simulink subsystem "IVTs"  (R2023b)
settings: Solver=VariableStepAuto  StartTime=0.0  StopTime=10.0  RelTol=1e-3
undefined symbols (not defined in the file): BServiceDisconnectNeg, BServiceDisconnectPos, tSimCont
settings Model: DataDictionary=Contactors_data.sldd  EnableAccessToBaseWorkspace=off  Creator=Elio  LastModifiedBy=Elio

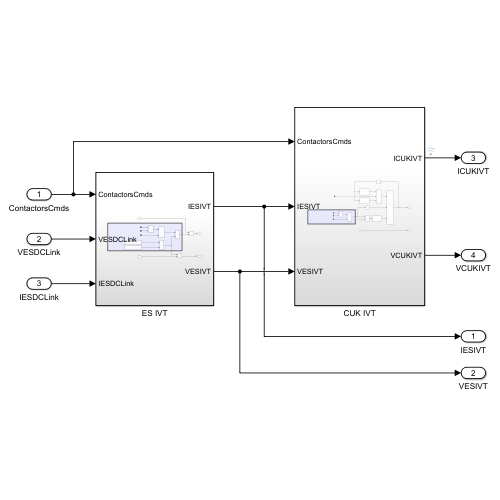
[thumbnail: Simulink's stored preview of the top-level diagram]
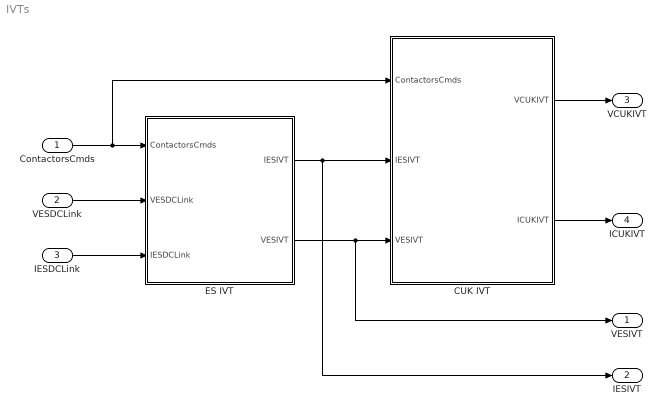
== system IVTs ==
  ContactorsCmds : Inport
  VESDCLink : Inport  Port=2
  IESDCLink : Inport  Port=3
  CUK IVT : Subsystem
  ES IVT : Subsystem
  VESIVT : Outport
  IESIVT : Outport  Port=2
  VCUKIVT : Outport  Port=3
  ICUKIVT : Outport  Port=4
  wires:
  ES IVT/1(IESIVT) -> IESIVT/1, CUK IVT/2(IESIVT)
  ES IVT/2(VESIVT) -> VESIVT/1, CUK IVT/3(VESIVT)
  CUK IVT/2(ICUKIVT) -> ICUKIVT/1
  CUK IVT/1(VCUKIVT) -> VCUKIVT/1
  ContactorsCmds/1 -> CUK IVT/1(ContactorsCmds), ES IVT/1(ContactorsCmds)
  VESDCLink/1 -> ES IVT/2(VESDCLink)
  IESDCLink/1 -> ES IVT/3(IESDCLink)

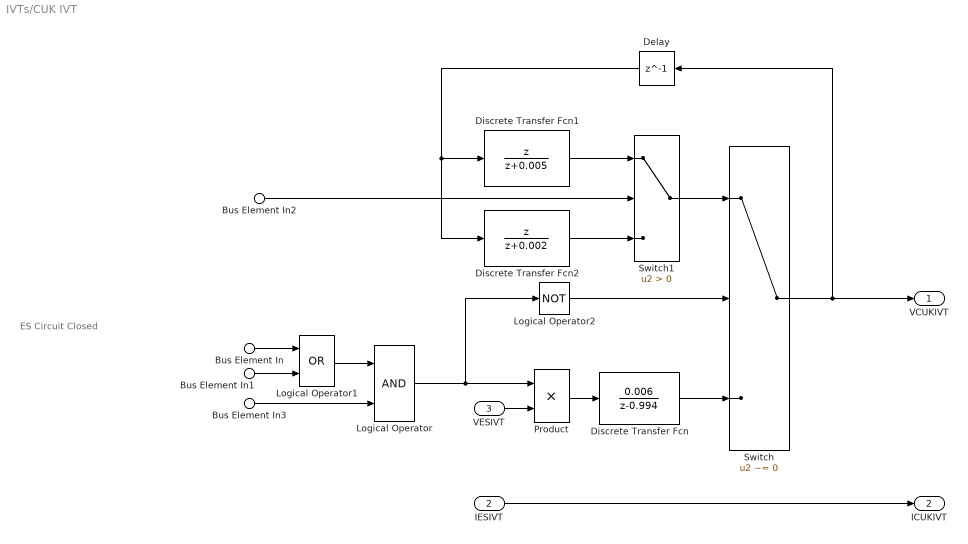
== system IVTs/CUK IVT ==
  note: ES Circuit Closed
  Bus Element In : Inport  PortName=ContactorsCmds  Element=BContPosRequested
  Bus Element In3 : Inport  PortName=ContactorsCmds  Element=BContNegRequested
  Bus Element In1 : Inport  PortName=ContactorsCmds  Element=BPrechargeRequested
  Bus Element In2 : Inport  PortName=ContactorsCmds  Element=BActiveDischargeRequested
  IESIVT : Inport  Port=2
  VESIVT : Inport  Port=3
  Delay : Delay  DelayLength=1
  Discrete Transfer Fcn : DiscreteTransferFcn  Numerator=[0.006]  Denominator=[1 -0.994]
  Discrete Transfer Fcn1 : DiscreteTransferFcn  Numerator=[1 0]  Denominator=[1 0.005]
  Discrete Transfer Fcn2 : DiscreteTransferFcn  Numerator=[1 0]  Denominator=[1 0.002]
  Logical Operator : Logic  AllPortsSameDT=off  OutDataTypeStr=boolean
  Logical Operator1 : Logic  Operator=OR  AllPortsSameDT=off  OutDataTypeStr=boolean
  Logical Operator2 : Logic  Operator=NOT  AllPortsSameDT=off  OutDataTypeStr=boolean
  Product : Product
  Switch : Switch  Criteria=u2 ~= 0  SaturateOnIntegerOverflow=off  InputSameDT=off
  Switch1 : Switch  Criteria=u2 > Threshold  SaturateOnIntegerOverflow=off  InputSameDT=off
  VCUKIVT : Outport
  ICUKIVT : Outport  Port=2
  wires:
  Switch/1 -> VCUKIVT/1, Delay/1
  Product/1 -> Discrete Transfer Fcn/1
  VESIVT/1 -> Product/2
  Bus Element In3/1 -> Logical Operator/2
  Logical Operator1/1 -> Logical Operator/1
  Bus Element In1/1 -> Logical Operator1/2
  Bus Element In/1 -> Logical Operator1/1
  Discrete Transfer Fcn/1 -> Switch/3
  Delay/1 -> Discrete Transfer Fcn1/1, Discrete Transfer Fcn2/1
  Bus Element In2/1 -> Switch1/2
  Logical Operator/1 -> Product/1, Logical Operator2/1
  Switch1/1 -> Switch/1
  Discrete Transfer Fcn1/1 -> Switch1/1
  Discrete Transfer Fcn2/1 -> Switch1/3
  Logical Operator2/1 -> Switch/2
  IESIVT/1 -> ICUKIVT/1

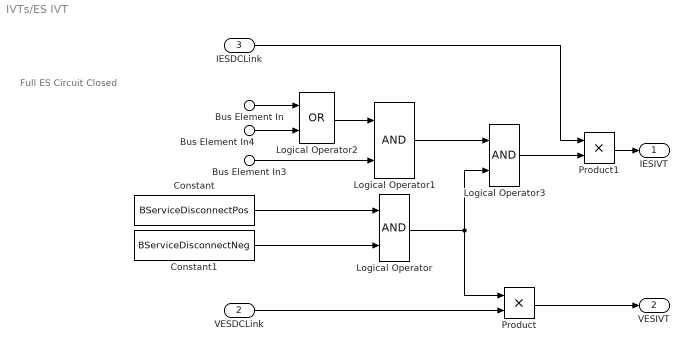
== system IVTs/ES IVT ==
  note: Full ES Circuit Closed
  Bus Element In : Inport  PortName=ContactorsCmds  Element=BContPosRequested
  Bus Element In3 : Inport  PortName=ContactorsCmds  Element=BContNegRequested
  Bus Element In4 : Inport  PortName=ContactorsCmds  Element=BPrechargeRequested
  VESDCLink : Inport  Port=2
  IESDCLink : Inport  Port=3
  Constant : Constant  Value=BServiceDisconnectPos  SampleTime=tSimCont
  Constant1 : Constant  Value=BServiceDisconnectNeg  SampleTime=tSimCont
  Logical Operator : Logic  AllPortsSameDT=off  OutDataTypeStr=boolean
  Logical Operator1 : Logic  AllPortsSameDT=off  OutDataTypeStr=boolean
  Logical Operator2 : Logic  Operator=OR  AllPortsSameDT=off  OutDataTypeStr=boolean
  Logical Operator3 : Logic  AllPortsSameDT=off  OutDataTypeStr=boolean
  Product : Product
  Product1 : Product
  IESIVT : Outport
  VESIVT : Outport  Port=2
  wires:
  VESDCLink/1 -> Product/2
  Constant/1 -> Logical Operator/1
  Logical Operator/1 -> Product/1, Logical Operator3/2
  Product/1 -> VESIVT/1
  Logical Operator2/1 -> Logical Operator1/1
  Bus Element In/1 -> Logical Operator2/1
  Bus Element In4/1 -> Logical Operator2/2
  Bus Element In3/1 -> Logical Operator1/2
  Logical Operator1/1 -> Logical Operator3/1
  Logical Operator3/1 -> Product1/2
  IESDCLink/1 -> Product1/1
  Product1/1 -> IESIVT/1
  Constant1/1 -> Logical Operator/2
